simulink model "hydraulic_system_characteristic"  (R2025b)
settings: Solver=VariableStepAuto  StartTime=0.0  StopTime=10  FixedStep=1e-5  RelTol=1e-4
model workspace (MAT data in the model file):
  GateChoice = "linear"
libraries: simulink x3
settings Model: Creator=LYG  LastModifiedBy=i336

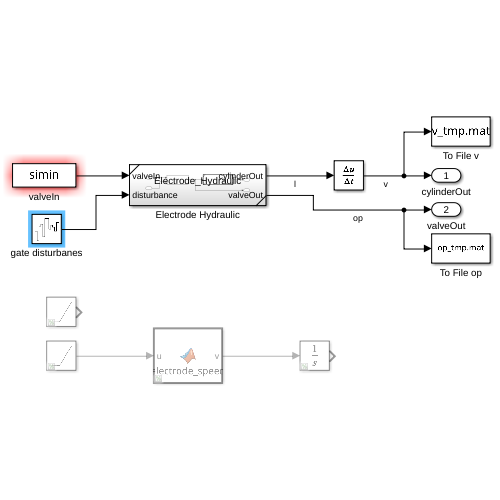
[thumbnail: Simulink's stored preview of the top-level diagram]
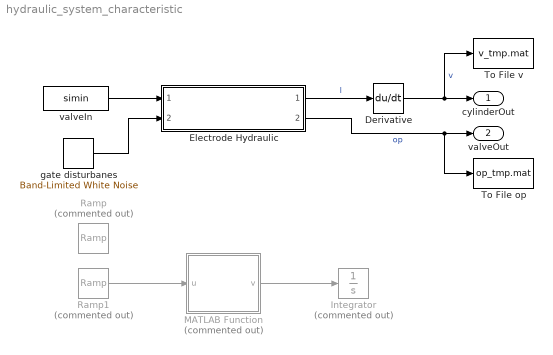
== system hydraulic_system_characteristic ==
  Derivative : Derivative
  Electrode Hydraulic : Subsystem  ReferencedSubsystem=Electrode_Hydraulic
  Integrator : Integrator  Commented=on  InitialCondition=0.5
  MATLAB Function : MATLAB Function  Commented=on  TreatAsAtomicUnit=on
  Ramp : simulink/Sources/Ramp  Commented=on  slope=0.2  start=0  InitialOutput=-1
  Ramp1 : simulink/Sources/Ramp  Commented=on  slope=5  start=0  InitialOutput=-15
  To File op : ToFile  Filename=op_tmp.mat  MatrixName=op  SaveFormat=Timeseries
  To File v : ToFile  Filename=v_tmp.mat  MatrixName=v  SaveFormat=Timeseries
  gate disturbanes : simulink/Sources/Band-Limited White Noise  Cov=2e-5  Ts=0.1  seed=[25584]
  valveIn : FromWorkspace  VariableName=simin
  cylinderOut : Outport
  valveOut : Outport  Port=2
  wires:
  Electrode Hydraulic/1 -> Derivative/1  "l"
  Derivative/1 -> To File v/1, cylinderOut/1  "v"
  Ramp1/1 -> MATLAB Function/1(u)
  MATLAB Function/1(v) -> Integrator/1
  Electrode Hydraulic/2 -> To File op/1, valveOut/1  "op"
  valveIn/1 -> Electrode Hydraulic/1
  gate disturbanes/1 -> Electrode Hydraulic/2

== matlab function hydraulic_system_characteristic/MATLAB Function ==
  data: u input; v output
function v = electrode_speed(u)
    % Parameters
    eps = 0.1;
    dl = -0.5; dr = 0.5;
    kl = 1.8; kr = 2.3;
    Sl = -9; Sr = 12;
    
    % voltage-speed characteristic
    v = zeros(1);
    softplus_l = eps * log(1 + exp((dl - u) / eps));
    softplus_r = eps * log(1 + exp((u - dr) / eps));
    w_soft = kr * softplus_r - kl * softplus_l;
    if u >= 0
        v(1) = Sr * tanh(w_soft / Sr);
    else
        v(1) = Sl * tanh(w_soft / Sl);
    end
end
